simulink model "lab6_sim3"  (R2024a)
settings: Solver=VariableStepAuto  StartTime=0.0  StopTime=10.0  RelTol=1e-3
libraries: simulink x1
settings Model: Creator=ventus  LastModifiedBy=ventus

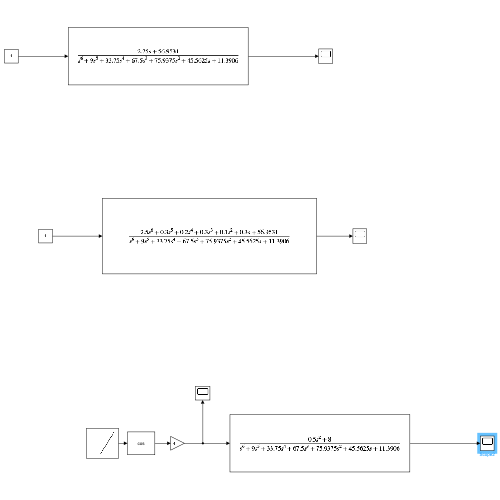
[thumbnail: Simulink's stored preview of the top-level diagram]
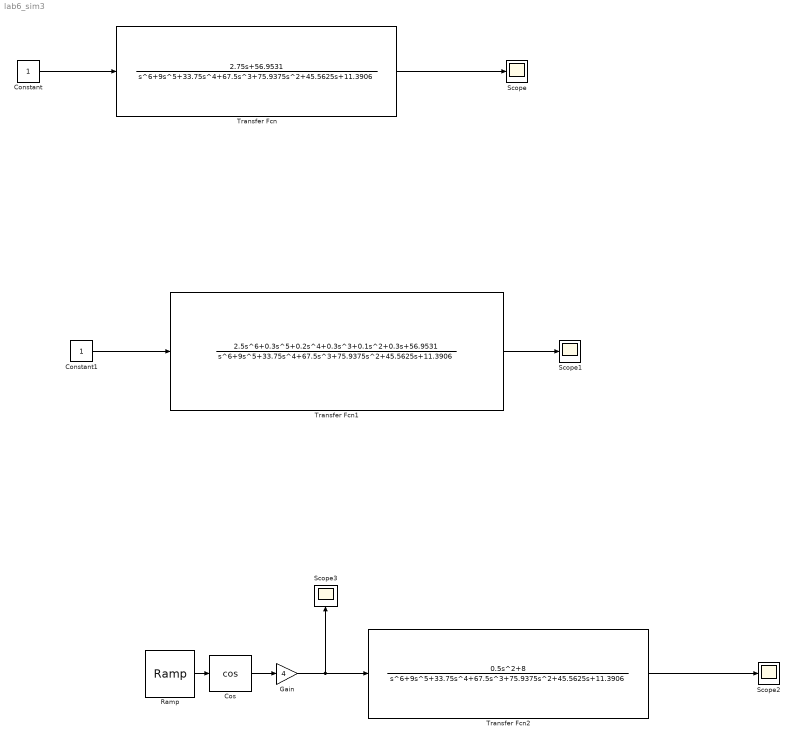
== system lab6_sim3 ==
  Constant : Constant
  Constant1 : Constant
  Cos : Trigonometry  Operator=cos
  Gain : Gain  Gain=4
  Ramp : simulink/Sources/Ramp  slope=4  start=0  InitialOutput=0
  Scope{,1..3} (4 alike) : Scope
  Transfer Fcn : TransferFcn  Numerator=[2.75 56.9531]  Denominator=|
      | [1
      |     9
      |    33.75
      |    67.5
      |    75.9375
      |    45.5625
      |    11.3906]
  Transfer Fcn1 : TransferFcn  Numerator=[2.5 0.3 0.2 0.3 0.1 0.3 56.9531]  Denominator=|
      | [1
      |     9
      |    33.75
      |    67.5
      |    75.9375
      |    45.5625
      |    11.3906]
  Transfer Fcn2 : TransferFcn  Numerator=[0.5 0 8]  Denominator=|
      | [1
      |     9
      |    33.75
      |    67.5
      |    75.9375
      |    45.5625
      |    11.3906]
  wires:
  Constant/1 -> Transfer Fcn/1
  Transfer Fcn/1 -> Scope/1
  Transfer Fcn1/1 -> Scope1/1
  Constant1/1 -> Transfer Fcn1/1
  Transfer Fcn2/1 -> Scope2/1
  Gain/1 -> Transfer Fcn2/1, Scope3/1
  Ramp/1 -> Cos/1
  Cos/1 -> Gain/1
